simulink library "csc_egt_egc_thruster_lib"  (R2014b)
settings: Solver=ode113  StartTime=0.0  StopTime=10.0  RelTol=1e-3
values from neighbouring files (symbols this model uses):
  egt_feed_pressure = 700    [csc_egt_egc_thruster_init.m]
  egt_g_times_isp = 120*9.80665    (= 1176.798)    [csc_egt_egc_thruster_init.m]
  egt_pc_to_thrust_offset = 37.1976248356    [csc_egt_egc_thruster_init.m]
  egt_pc_to_thrust_slope = 1.32839171615    [csc_egt_egc_thruster_init.m]
  tpl_egc_chamber_pressure_to_thrust = [ EGC_Pc' EGC_Thrust']    [csc_egt_egc_thruster_init.m]
  tpl_egc_throttle_to_mdot_gain = 1.0    (= 1)    [csc_egt_egc_thruster_init.m]
  tpl_egc_throttle_to_thrust = [                                  0.0     0        ;                                  0.2     1323.761 ;                                  0.25	1489.577 ;                                  0.3     1630.213 ;                                  0.35	1748.769 ;                                  0.4     1848.346 ;                                  0.45	1932.047 ;                                  0.5     20 ...(+513 chars)    [csc_egt_egc_thruster_init.m]
  tpl_egc_throttle_to_thrust_gain = 1.0    (= 1)    [csc_egt_egc_thruster_init.m]
undefined symbols (not defined in the file or in its folder): mpl_htp_mass_initial
libraries: simulink x4, csu_spv_simulated_press_valves_lib x4, util_common_lib x4, util_event_lib x2, util_info_lib x1, util_thruster_lib x1
settings Model: Creator=Jim Kaidy  LastModifiedBy=escrane

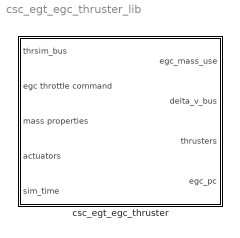
== system csc_egt_egc_thruster_lib ==
  csc_egt_egc_thruster : Subsystem

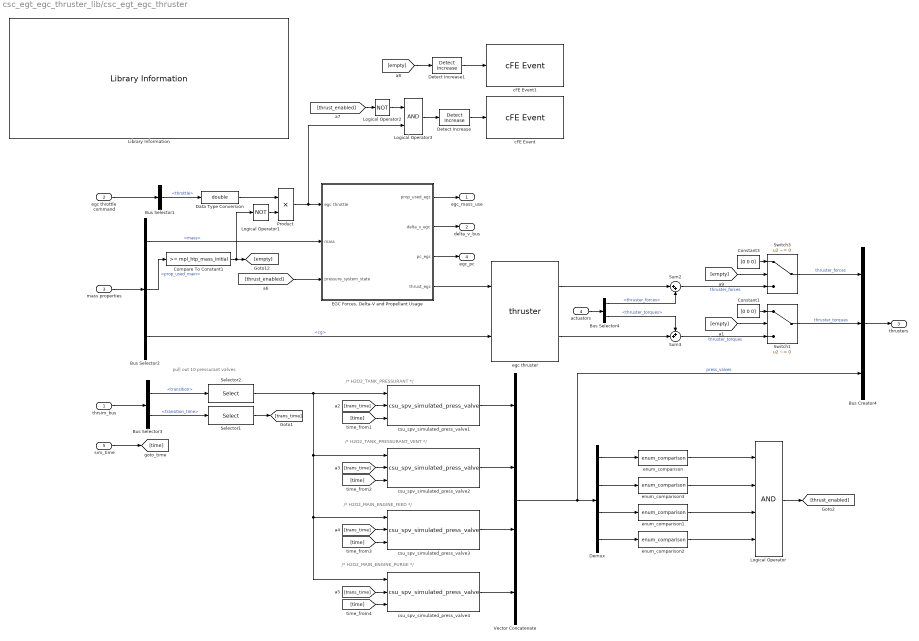
== system csc_egt_egc_thruster_lib/csc_egt_egc_thruster ==
  note: pull out 10 pressurant valves
  note: /* H2O2_TANK_PRESSURANT */
  note: /* H2O2_TANK_PRESSURANT_VENT */
  note: /* H2O2_MAIN_ENGINE_FEED */
  note: /* H2O2_MAIN_ENGINE_PURGE */
  thrsim_bus : Inport
  egc throttle command : Inport  Port=2
  mass properties : Inport  Port=3
  actuators : Inport  Port=4
  sim_time : Inport  Port=5
  Bus Creator4 : BusCreator  Inputs=3
  Bus Selector1 : BusSelector  OutputSignals=throttle
  Bus Selector2 : BusSelector  OutputSignals=mass,prop_used_main,cg
  Bus Selector3 : BusSelector  OutputSignals=transition,transition_time
  Bus Selector4 : BusSelector  OutputSignals=thruster_forces,thruster_torques
  Compare To Constant1 : simulink/Logic and Bit Operations/Compare To Constant  relop=>=  const=mpl_htp_mass_initial  OutDataTypeStr=boolean
  Constant1 : Constant  Value=[0 0 0]
  Constant3 : Constant  Value=[0 0 0]
  Data Type Conversion : DataTypeConversion  OutDataTypeStr=double
  Demux : Demux
  Detect Increase : simulink/Logic and Bit Operations/Detect Increase  vinit=0.0  InputProcessing=Inherited  OutDataTypeStr=boolean
  Detect Increase1 : simulink/Logic and Bit Operations/Detect Increase  vinit=0.0  InputProcessing=Inherited  OutDataTypeStr=boolean
  "EGC Forces, Delta-V and Propellant Usage" : Subsystem
  Library Information : util_info_lib/Library Information  owner='NONE'
  Logical Operator : Logic  Inputs=4  AllPortsSameDT=off  OutDataTypeStr=boolean
  Logical Operator1 : Logic  Operator=NOT  AllPortsSameDT=off  OutDataTypeStr=boolean
  Logical Operator2 : Logic  Operator=NOT  AllPortsSameDT=off  OutDataTypeStr=boolean
  Logical Operator3 : Logic  AllPortsSameDT=off  OutDataTypeStr=boolean
  Product : Product
  Selector1 : Selector  InputPortWidth=22  Indices=[13:22]
  Selector2 : Selector  InputPortWidth=22  Indices=[13:22]
  Sum2 : Sum  Inputs=|++
  Sum3 : Sum  Inputs=++|
  Switch1 : Switch  Criteria=u2 ~= 0
  Switch3 : Switch  Criteria=u2 ~= 0
  Vector Concatenate : Concatenate  NumInputs=4
  cFE Event : util_event_lib/cFE Event  event_message='EGC commanded with bad latch valve config. No thrust.'  event_id=22  event_severity=INFORMATION  event_use_enums=off  event_enum_types={}
  cFE Event1 : util_event_lib/cFE Event  event_message='Out of HTP!'  event_id=22  event_severity=INFORMATION  event_use_enums=off  event_enum_types={}
  csu_spv_simulated_press_valve1 : csu_spv_simulated_press_valves_lib/csu_spv_simulated_press_valve  thruster_idx=1  num_thrusters=10  energized_value=1  deenergized_value=0
  csu_spv_simulated_press_valve2 : csu_spv_simulated_press_valves_lib/csu_spv_simulated_press_valve  thruster_idx=2  num_thrusters=10  energized_value=0  deenergized_value=1
  csu_spv_simulated_press_valve3 : csu_spv_simulated_press_valves_lib/csu_spv_simulated_press_valve  thruster_idx=4  num_thrusters=10  energized_value=1  deenergized_value=0
  csu_spv_simulated_press_valve4 : csu_spv_simulated_press_valves_lib/csu_spv_simulated_press_valve  thruster_idx=5  num_thrusters=10  energized_value=1  deenergized_value=0
  egc thruster : util_thruster_lib/thruster  Thruster_Position=tfl_thruster_egc_position  Thruster_Orientation=tfl_thruster_egc_orientation
  enum_comparison{,1..3} (4 alike) : util_common_lib/enum_comparison  comparison_type===
  egc_mass_use : Outport
  delta_v_bus : Outport  Port=2
  thrusters : Outport  Port=3
  egc_pc : Outport  Port=4
  wires:
  Detect Increase1/1 -> cFE Event1/1
  [empty] -> Detect Increase1/1
  Detect Increase/1 -> cFE Event/1
  [thrust_enabled] -> Logical Operator2/1
  Logical Operator2/1 -> Logical Operator3/1
  Logical Operator3/1 -> Detect Increase/1
  Demux/4 -> enum_comparison2/1
  Demux/3 -> enum_comparison1/1
  Demux/2 -> enum_comparison3/1
  Demux/1 -> enum_comparison/1
  Vector Concatenate/1 -> Demux/1, Bus Creator4/3  "press_valves"
  Logical Operator1/1 -> Product/2
  Bus Selector2/2 -> Compare To Constant1/1  "<prop_used_main>"
  [thrust_enabled] -> "EGC Forces, Delta-V and Propellant Usage"/3(pressure_system_state)
  Logical Operator/1 -> [thrust_enabled]
  enum_comparison2/1 -> Logical Operator/4
  enum_comparison1/1 -> Logical Operator/3
  enum_comparison3/1 -> Logical Operator/2
  enum_comparison/1 -> Logical Operator/1
  csu_spv_simulated_press_valve2/1 -> Vector Concatenate/2
  csu_spv_simulated_press_valve4/1 -> Vector Concatenate/4
  csu_spv_simulated_press_valve3/1 -> Vector Concatenate/3
  csu_spv_simulated_press_valve1/1 -> Vector Concatenate/1
  Selector2/1 -> csu_spv_simulated_press_valve1/1, csu_spv_simulated_press_valve2/1, csu_spv_simulated_press_valve3/1, csu_spv_simulated_press_valve4/1
  [time] -> csu_spv_simulated_press_valve4/3
  [trans_time] -> csu_spv_simulated_press_valve4/2
  [time] -> csu_spv_simulated_press_valve3/3
  [trans_time] -> csu_spv_simulated_press_valve3/2
  [time] -> csu_spv_simulated_press_valve2/3
  [trans_time] -> csu_spv_simulated_press_valve2/2
  [time] -> csu_spv_simulated_press_valve1/3
  sim_time/1 -> [time]
  [trans_time] -> csu_spv_simulated_press_valve1/2
  Bus Selector3/2 -> Selector1/1  "<transition_time>"
  Bus Selector3/1 -> Selector2/1  "<transition>"
  Selector1/1 -> [trans_time]
  thrsim_bus/1 -> Bus Selector3/1
  [empty] -> Switch1/2
  [empty] -> Switch3/2
  Compare To Constant1/1 -> Logical Operator1/1, [empty]
  Constant1/1 -> Switch1/1
  Bus Selector1/1 -> Data Type Conversion/1  "<throttle>"
  "EGC Forces, Delta-V and Propellant Usage"/1(prop_used_egc) -> egc_mass_use/1
  "EGC Forces, Delta-V and Propellant Usage"/2(delta_v_egc) -> delta_v_bus/1
  "EGC Forces, Delta-V and Propellant Usage"/4(thrust_egc) -> egc thruster/1
  mass properties/1 -> Bus Selector2/1
  Bus Selector2/1 -> "EGC Forces, Delta-V and Propellant Usage"/2(mass)  "<mass>"
  Bus Selector2/3 -> egc thruster/2  "<cg>"
  Bus Selector4/1 -> Sum2/2  "<thruster_forces>"
  actuators/1 -> Bus Selector4/1
  egc thruster/1 -> Sum2/1
  egc thruster/2 -> Sum3/2
  Bus Selector4/2 -> Sum3/1  "<thruster_torques>"
  Bus Creator4/1 -> thrusters/1
  Sum3/1 -> Switch1/3  "thruster_torques"
  Sum2/1 -> Switch3/3  "thruster_forces"
  Data Type Conversion/1 -> Product/1
  egc throttle command/1 -> Bus Selector1/1
  Constant3/1 -> Switch3/1
  Switch3/1 -> Bus Creator4/1  "thruster_forces"
  Switch1/1 -> Bus Creator4/2  "thruster_torques"
  Product/1 -> "EGC Forces, Delta-V and Propellant Usage"/1(egc throttle), Logical Operator3/2
  "EGC Forces, Delta-V and Propellant Usage"/3(pc_egc) -> egc_pc/1

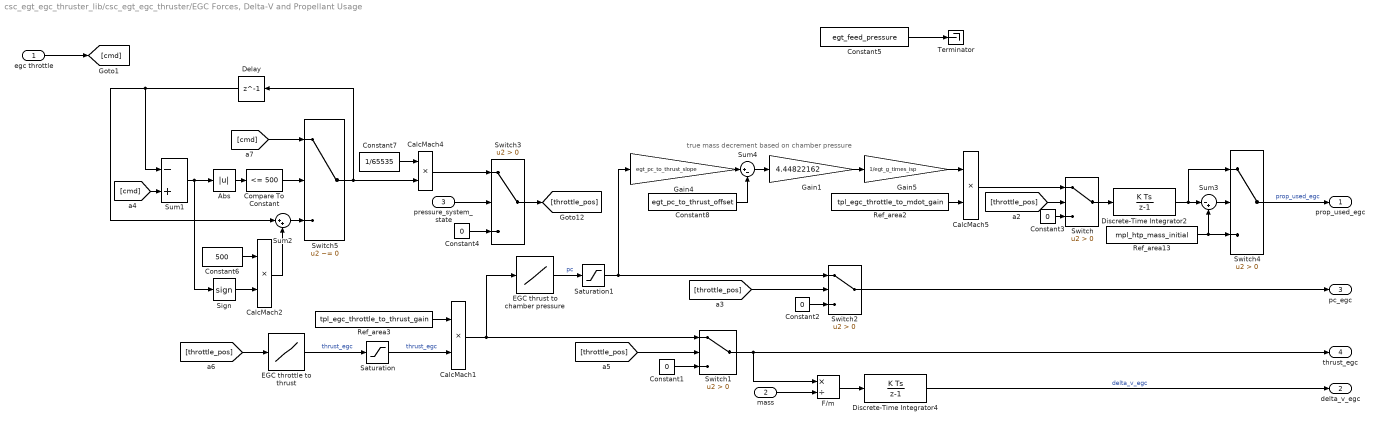
== system csc_egt_egc_thruster_lib/csc_egt_egc_thruster/EGC Forces, Delta-V and Propellant Usage ==
  note: true mass decrement based on chamber pressure
  egc throttle : Inport
  mass : Inport  Port=2
  pressure_system_state : Inport  Port=3
  Abs : Abs
  CalcMach{1..2,4..5} (4 alike) : Product  SaturateOnIntegerOverflow=on  OutDataTypeStr=Inherit: Same as first input
  Compare To Constant : simulink/Logic and Bit Operations/Compare To Constant  relop=<=  const=500  OutDataTypeStr=boolean
  Constant{1..4} (4 alike) : Constant  Value=0
  Constant5 : Constant  Value=egt_feed_pressure
  Constant6 : Constant  Value=500
  Constant7 : Constant  Value=1/65535
  Constant8 : Constant  Value=egt_pc_to_thrust_offset  OutDataTypeStr=double
  Delay : Delay  DelayLength=1
  Discrete-Time Integrator2 : DiscreteIntegrator  gainval=1  SampleTime=-1
  Discrete-Time Integrator4 : DiscreteIntegrator  gainval=1  SampleTime=-1
  "EGC thrust to chamber pressure " : Lookup  InputValues=tpl_egc_chamber_pressure_to_thrust(:,2)  Table=tpl_egc_chamber_pressure_to_thrust(:,1)
  EGC throttle to thrust : Lookup  InputValues=tpl_egc_throttle_to_thrust(:,1)  Table=tpl_egc_throttle_to_thrust(:,2)
  F/m : Product  Inputs=*/
  Gain1 : Gain  Gain=4.44822162
  Gain4 : Gain  Gain=egt_pc_to_thrust_slope
  Gain5 : Gain  Gain=1/egt_g_times_isp
  Ref_area13 : Constant  Value=mpl_htp_mass_initial
  Ref_area2 : Constant  Value=tpl_egc_throttle_to_mdot_gain
  Ref_area3 : Constant  Value=tpl_egc_throttle_to_thrust_gain
  Saturation : Saturate  UpperLimit=3000  LowerLimit=0
  Saturation1 : Saturate  UpperLimit=600  LowerLimit=0
  Sign : Signum
  Sum1 : Sum  Inputs=-+
  Sum2 : Sum  Inputs=|++
  Sum3 : Sum  Inputs=|-+
  Sum4 : Sum  Inputs=|+-
  Switch{,1..4} (5 alike) : Switch  Criteria=u2 > Threshold
  Switch5 : Switch  Criteria=u2 ~= 0
  Terminator : Terminator
  prop_used_egc : Outport
  delta_v_egc : Outport  Port=2
  pc_egc : Outport  Port=3
  thrust_egc : Outport  Port=4
  wires:
  CalcMach5/1 -> Switch/1
  Ref_area2/1 -> CalcMach5/2
  Saturation1/1 -> Gain4/1, Switch2/1
  EGC throttle to thrust/1 -> Saturation/1  "thrust_egc"
  [throttle_pos] -> EGC throttle to thrust/1
  Switch3/1 -> [throttle_pos]
  Constant8/1 -> Sum4/2
  Gain4/1 -> Sum4/1
  Gain1/1 -> Gain5/1
  Sum4/1 -> Gain1/1
  "EGC thrust to chamber pressure "/1 -> Saturation1/1  "pc"
  Constant7/1 -> CalcMach4/1
  CalcMach4/1 -> Switch3/1
  Sign/1 -> CalcMach2/2
  Constant6/1 -> CalcMach2/1
  CalcMach2/1 -> Sum2/2
  Sum2/1 -> Switch5/3
  Switch5/1 -> Delay/1, CalcMach4/2
  [cmd] -> Switch5/1
  [cmd] -> Sum1/2
  Compare To Constant/1 -> Switch5/2
  Abs/1 -> Compare To Constant/1
  Sum1/1 -> Abs/1, Sign/1
  Delay/1 -> Sum2/1, Sum1/1
  egc throttle/1 -> [cmd]
  Ref_area3/1 -> CalcMach1/1
  Gain5/1 -> CalcMach5/1
  Constant5/1 -> Terminator/1
  Ref_area13/1 -> Sum3/2, Switch4/3
  Discrete-Time Integrator2/1 -> Sum3/1, Switch4/1
  Sum3/1 -> Switch4/2
  Constant4/1 -> Switch3/3
  pressure_system_state/1 -> Switch3/2
  Discrete-Time Integrator4/1 -> delta_v_egc/1  "delta_v_egc"
  Switch4/1 -> prop_used_egc/1  "prop_used_egc"
  F/m/1 -> Discrete-Time Integrator4/1
  mass/1 -> F/m/2
  Constant3/1 -> Switch/3
  [throttle_pos] -> Switch/2
  Switch/1 -> Discrete-Time Integrator2/1
  Switch1/1 -> thrust_egc/1, F/m/1
  Constant1/1 -> Switch1/3
  [throttle_pos] -> Switch1/2
  Saturation/1 -> CalcMach1/2  "thrust_egc"
  Constant2/1 -> Switch2/3
  [throttle_pos] -> Switch2/2
  Switch2/1 -> pc_egc/1
  CalcMach1/1 -> "EGC thrust to chamber pressure "/1, Switch1/1
